simulink model "krzywe_pogodowe_obliczanie_zapotrzebowania"  (R2021b)
settings: Solver=VariableStepAuto  StartTime=0.0  StopTime=10.0  RelTol=1e-3
undefined symbols (not defined in the file): ap, az, bp, bz, cpw, fmgN
settings Model: Creator=adams  LastModifiedBy=adams

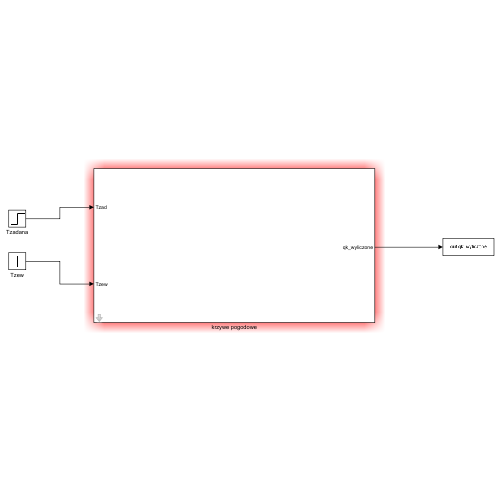
[thumbnail: Simulink's stored preview of the top-level diagram]
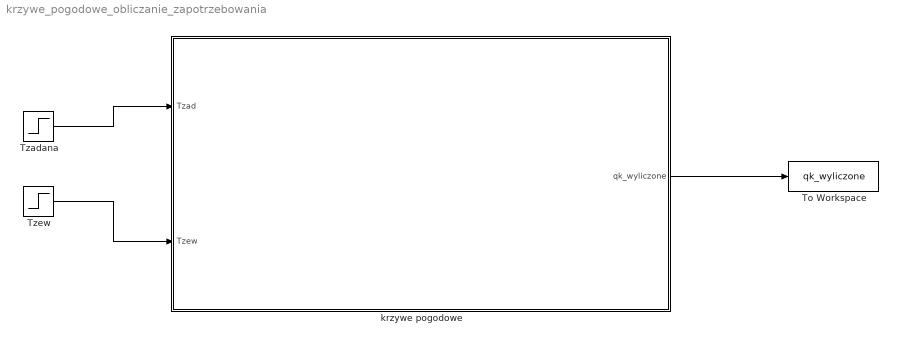
== system krzywe_pogodowe_obliczanie_zapotrzebowania ==
  To Workspace : ToWorkspace  VariableName=qk_wyliczone  SampleTime=-1
  Tzadana : Step  SampleTime=0
  Tzew : Step  SampleTime=0
  krzywe pogodowe : Subsystem  mask{az=az, bz=bz, ap=ap, bp=bp, cpw=cpw, fmgN=fmgN}
  wires:
  Tzadana/1 -> krzywe pogodowe/1(Tzad)
  Tzew/1 -> krzywe pogodowe/2(Tzew)
  krzywe pogodowe/1(qk_wyliczone) -> To Workspace/1

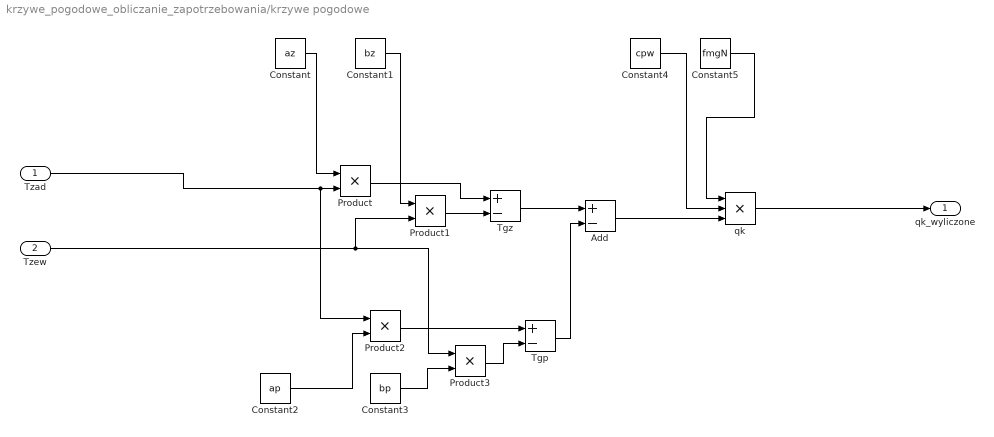
== system krzywe_pogodowe_obliczanie_zapotrzebowania/krzywe pogodowe ==
  Tzad : Inport
  Tzew : Inport  Port=2
  Add : Sum  Inputs=+-
  Constant : Constant  Value=az
  Constant1 : Constant  Value=bz
  Constant2 : Constant  Value=ap
  Constant3 : Constant  Value=bp
  Constant4 : Constant  Value=cpw
  Constant5 : Constant  Value=fmgN
  Product{,1..3} (4 alike) : Product
  Tgp : Sum  Inputs=+-
  Tgz : Sum  Inputs=+-
  qk : Product  Inputs=3
  qk_wyliczone : Outport
  wires:
  Add/1 -> qk/3
  Product/1 -> Tgz/1
  Constant1/1 -> Product1/1
  Product1/1 -> Tgz/2
  Product3/1 -> Tgp/2
  Product2/1 -> Tgp/1
  Tzad/1 -> Product2/1, Product/2
  Tgz/1 -> Add/1
  Constant3/1 -> Product3/2
  Constant4/1 -> qk/2
  Tzew/1 -> Product3/1, Product1/2
  Constant5/1 -> qk/1
  Tgp/1 -> Add/2
  Constant2/1 -> Product2/2
  Constant/1 -> Product/1
  qk/1 -> qk_wyliczone/1
